simulink model "motorPID_tuning_speedLoop"  (R2021b)
settings: Solver=FixedStepAuto  StartTime=0.0  StopTime=600  FixedStep=0.004  RelTol=1e-3  EnableMultiTasking=on
settings Model: Creator=The MathWorks, Inc.  LastModifiedBy=kboxi
settings SolverCC: ConcurrentTasks=on  AlgebraicLoopSolver=TrustRegion  PositivePriorityOrder=on
settings DataIOCC: ReturnWorkspaceOutputs=off
settings OptimizationCC: EnhancedBackFolding=on  PassReuseOutputArgsThreshold=0  MaxStackSize=64  OptimizeBlockOrder=speed  DifferentSizesBufferReuse=on  OptimizationCustomize=off
settings DebuggingCC: ParameterTunabilityLossMsg=error  SFMachineParentedDataDiag=warning
settings HardwareCC: ProdBitPerPointer=32  ProdBitPerSizeT=32  ProdBitPerPtrDiffT=32  ProdLargestAtomicInteger=Long  ProdLargestAtomicFloat=Double  ProdWordSize=32  ProdLongLongMode=on  ProdHWDeviceType=ARM Compatible->ARM Cortex  UseEmbeddedCoderFeatures=off
settings RTWCC: Description=Embedded Coder  SystemTargetFile=ert.tlc  HardwareBoard=Raspberry Pi  TLCOptions="-aInlineSetEventsForThisBaseRateFcn=TLC_FALSE -aSuppressMultiTaskScheduler=TLC_FALSE  -aRateBasedStepFcn=0"  TemplateMakefile=ert_default_tmf  Toolchain=GNU GCC Embedded Linux  BuildConfiguration=Faster Runs
settings CodeAppCC: ForceParamTrailComments=on  OperatorAnnotations=on
settings ERTTargetCC: ERTCustomFileBanners=off  SupportContinuousTime=on  SupportNonInlinedSFcns=on  RemoveResetFunc=off  SupportVariableSizeSignals=on  ModelStepFunctionPrototypeControlCompliant=off  ExtModeTransport=2  ExtModeStaticAlloc=on  ExtModeMexFile=ext_xcp  ExtModeIntrfLevel=Level2 - Open

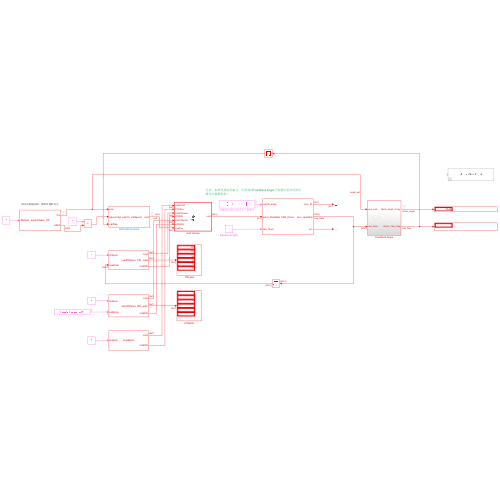
[thumbnail: Simulink's stored preview of the top-level diagram]
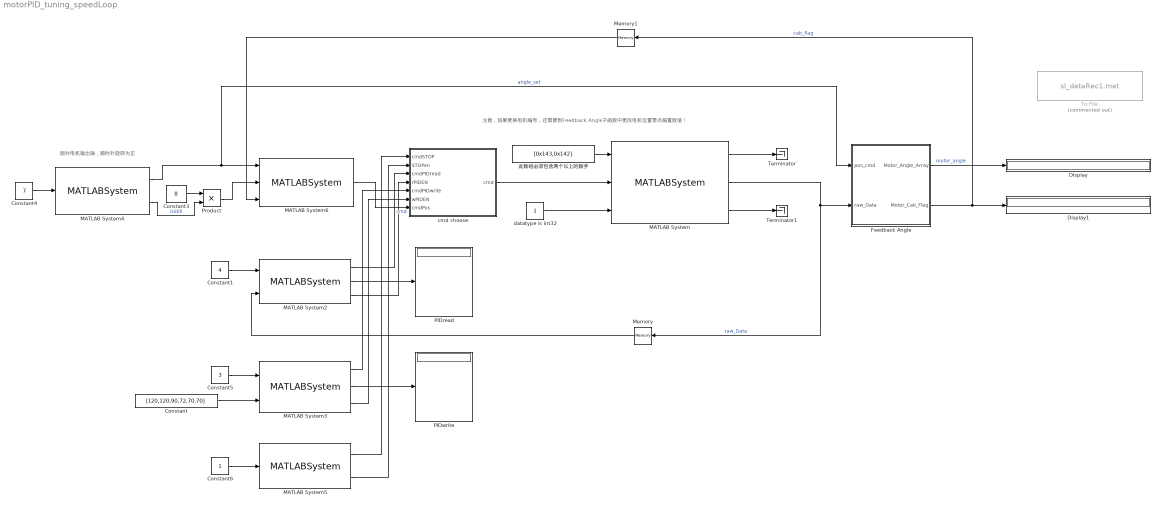
== system motorPID_tuning_speedLoop ==
  note: 注意，如果更换电机编号，还需要到Feedback Angle子函数中更改电机位置零点偏置数值！
  note: 面对电机输出轴，顺时针旋转为正
  Constant : Constant  Value=[120,120,90,72,70,70]
  Constant1 : Constant  Value=4  OutDataTypeStr=double
  Constant3 : Constant  Value=8
  Constant4 : Constant  Value=7
  Constant5 : Constant  Value=3  OutDataTypeStr=double
  Constant6 : Constant  OutDataTypeStr=double
  Display : Display
  Display1 : Display
  Feedback Angle : Subsystem
  MATLAB System : MATLABSystem  System=canSendRecv  canPort=can1
      mask Type: canSendRecv
      mask Display:
      | disp('CAN_Driver');
      | port_label('input',1,'canID_array');
      | port_label('input',2,'send_RawData');
      | port_label('input',3,'dev_Num');
      | port_label('output',1,'recv_ID');
      | port_label('output',2,'recv_rawData');
      | port_label('output',3,'err');
  MATLAB System2 : MATLABSystem  System=readPIDpara  SimulateUsing=Code generation
      mask Type: readPIDpara
      mask Display:
      | disp('readPIDpara');
      | port_label('input',1,'EnNum');
      | port_label('input',2,'rawData');
      | port_label('output',1,'cmd');
      | port_label('output',2,'PID_read');
      | port_label('output',3,'cmdEN');
  MATLAB System3 : MATLABSystem  System=writePIDpara  toRAM=0  SimulateUsing=Code generation
      mask Type: writePIDpara
      mask Display:
      | disp('writePIDpara');
      | port_label('input',1,'EnNum');
      | port_label('input',2,'pidArray');
      | port_label('output',1,'cmd');
      | port_label('output',2,'PID_write');
      | port_label('output',3,'cmdEN');
  MATLAB System4 : MATLABSystem  System=squareWave_OP  tHigh=0.5  tLow=0.5  Amp=10  SampleTime=0.004  OffsetTime=0  TickTime=0  SimulateUsing=Code generation
      mask Type: squareWave_OP
      mask Display:
      | disp('squareWave_OP');
      | port_label('input',1,'ENNum');
      | port_label('output',1,'Tra');
      | port_label('output',2,'isStill');
  MATLAB System5 : MATLABSystem  System=stopMotor  SimulateUsing=Code generation
      mask Type: stopMotor
      mask Display:
      | disp('stopMotor');
      | port_label('input',1,'EnNum');
      | port_label('output',1,'cmd');
      | port_label('output',2,'cmdEN');
  MATLAB System6 : MATLABSystem  System=Sgl_posCtr_viaSpeed  dt=0.004  SimulateUsing=Code generation
      mask Type: Sgl_posCtr_viaSpeed
      mask Display:
      | disp('Sgl_posCtr_viaSpeed');
      | port_label('input',1,'pos');
      | port_label('input',2,'speed');
      | port_label('input',3,'calFlag');
      | port_label('output',1,'cmd');
  Memory : Memory  InitialCondition=zeros(32,1)
  Memory1 : Memory
  PIDread : Display
  PIDwrite : Display
  Product : Product
  Terminator : Terminator
  Terminator1 : Terminator
  To File : ToFile  Commented=on  Filename=sl_dataRec1.mat  MatrixName=MotorAngle_cab_Encoder
  cmd choose : MATLAB Function  TreatAsAtomicUnit=on
  datatype is int32 : Constant  OutDataTypeStr=int32
  此数组必须包含两个以上的数字 : Constant  Value=[0x143,0x142]
  wires:
  此数组必须包含两个以上的数字/1 -> MATLAB System/1
  datatype is int32/1 -> MATLAB System/3
  MATLAB System/1 -> Terminator/1
  MATLAB System/3 -> Terminator1/1
  MATLAB System/2 -> Memory/1, Feedback Angle/2(raw_Data)  "raw_Data"
  Constant4/1 -> MATLAB System4/1
  MATLAB System4/1 -> MATLAB System6/1, Feedback Angle/1(pos_cmd)  "angle_set"
  Feedback Angle/1(Motor_Angle_Array) -> Display/1  "motor_angle"
  Feedback Angle/2(Motor_Cab_Flag) -> Memory1/1, Display1/1  "cab_flag"
  Constant3/1 -> Product/1
  Product/1 -> MATLAB System6/2
  MATLAB System4/2 -> Product/2  "isStill"
  Memory1/1 -> MATLAB System6/3
  Constant1/1 -> MATLAB System2/1
  Memory/1 -> MATLAB System2/2
  cmd choose/1(cmd) -> MATLAB System/2
  MATLAB System6/1 -> cmd choose/7(cmdPos)  "cmd"
  MATLAB System2/1 -> cmd choose/3(cmdPIDread)
  MATLAB System2/3 -> cmd choose/4(rPIDEN)
  MATLAB System2/2 -> PIDread/1
  MATLAB System3/2 -> PIDwrite/1
  MATLAB System3/1 -> cmd choose/5(cmdPIDwrite)
  MATLAB System3/3 -> cmd choose/6(wPIDEN)
  Constant5/1 -> MATLAB System3/1
  Constant/1 -> MATLAB System3/2
  Constant6/1 -> MATLAB System5/1
  MATLAB System5/1 -> cmd choose/1(cmdSTOP)
  MATLAB System5/2 -> cmd choose/2(STOPen)

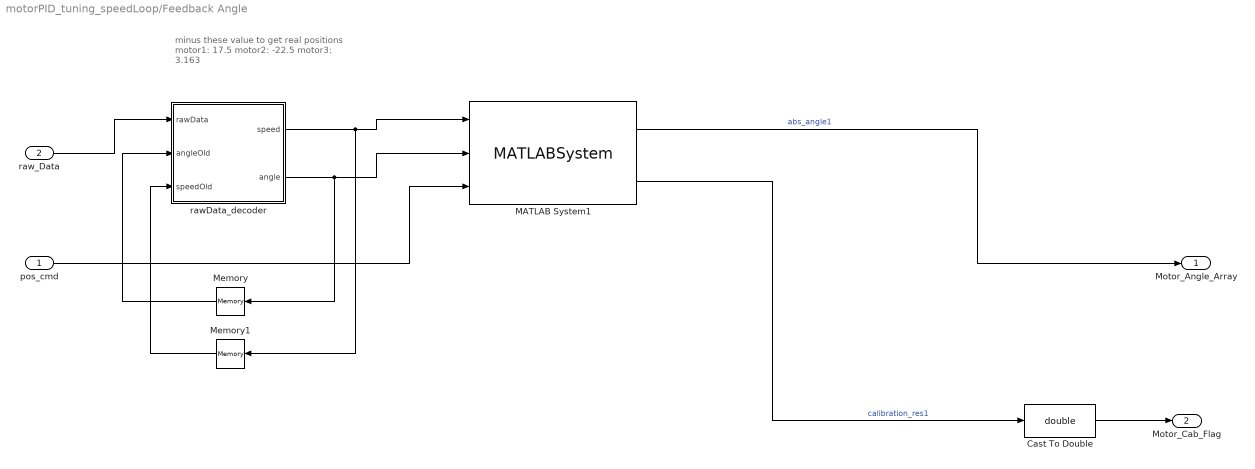
== system motorPID_tuning_speedLoop/Feedback Angle ==
  note: minus these value to get real positions
      | motor1: 17.5
      | motor2: -22.5
      | motor3: 3.163
  pos_cmd : Inport
  raw_Data : Inport  Port=2
  Cast To Double : DataTypeConversion  OutDataTypeStr=double
  MATLAB System1 : MATLABSystem  System=MotorAngle  angleOff=22.5  SimulateUsing=Code generation
      mask Type: MotorAngle
      mask Display:
      | disp('MotorAngle');
      | port_label('input',1,'speed');
      | port_label('input',2,'sgl_angle');
      | port_label('input',3,'pos_des');
      | port_label('output',1,'abs_angle');
      | port_label('output',2,'calibration');
  Memory : Memory
  Memory1 : Memory
  rawData_decoder : MATLAB Function  TreatAsAtomicUnit=on
  Motor_Angle_Array : Outport
  Motor_Cab_Flag : Outport  Port=2
  wires:
  raw_Data/1 -> rawData_decoder/1(rawData)
  rawData_decoder/2(angle) -> Memory/1, MATLAB System1/2
  MATLAB System1/1 -> Motor_Angle_Array/1  "abs_angle1"
  rawData_decoder/1(speed) -> Memory1/1, MATLAB System1/1
  MATLAB System1/2 -> Cast To Double/1  "calibration_res1"
  Cast To Double/1 -> Motor_Cab_Flag/1
  pos_cmd/1 -> MATLAB System1/3
  Memory/1 -> rawData_decoder/2(angleOld)
  Memory1/1 -> rawData_decoder/3(speedOld)

== matlab function motorPID_tuning_speedLoop/cmd choose ==
  data: cmdSTOP input; cmd output; STOPen input; cmdPIDread input; rPIDEN input; cmdPIDwrite input; wPIDEN input; cmdPos input
function cmd = fcn(cmdSTOP,STOPen,cmdPIDread,rPIDEN,cmdPIDwrite,wPIDEN,cmdPos)
if STOPen>0.5
    cmd=cmdSTOP;
    return;
end
if rPIDEN>0.5
    cmd=cmdPIDread;
    return;
end
if wPIDEN>0.5
    cmd=cmdPIDwrite;
    return;
end
cmd=cmdPos;

== matlab function motorPID_tuning_speedLoop/Feedback Angle/rawData_decoder ==
  data: speed output size=[1,1]; rawData input uint8; angle output size=[1,1]; angleOld input size=[1,1]; speedOld input size=[1,1]
function [speed,angle] = fcn(rawData,angleOld,speedOld)
% angle : single loop position, degree
% speed : speed after the reducer, degree per second

if (rawData(1)==0xa4 || rawData(1)==0xa2)
idx=1;
angle = double(typecast(rawData(idx+6:idx+7),'uint16'))/65535*360;
speed = double(typecast(rawData(idx+4:idx+5),'int16'))/6;
else
    angle=angleOld;
    speed=speedOld;
end
